simulink subsystem "sscfluids_ev_thermal_management"  (R2021b)
settings: Solver=VariableStepAuto  StartTime=0.0  StopTime=10.0  RelTol=1e-3
undefined symbols (not defined in the file): BattTempInit, bulb, cabin_duct_area, cabin_T_init, chiller_area_primary, chiller_N_baffles, chiller_N_tubes, chiller_tube_D, chiller_tube_L, chiller_wall_conductivity, chiller_wall_thickness, compressor_rpm_LUT, condenser_air_area_flow, condenser_air_area_primary, condenser_W, condenser_wall_conductivity, condenser_wall_thickness, coolant_channel_D, coolant_pipe_D, coolant_T_init, coolant_tank_area, coolant_tank_volume, coolant_valve_D_ratio_max, coolant_valve_D_ratio_min, coolant_valve_displacement, evaporator_air_area_flow, evaporator_air_area_primary, evaporator_W, evaporator_wall_conductivity, evaporator_wall_thickness, fan_area, outlet, pump_displacement, pump_speed_max, radiator_air_area_flow, radiator_air_area_primary, radiator_W, radiator_wall_conductivity, radiator_wall_thickness, refrigerant_alpha_init, refrigerant_pipe_D
libraries: fl_lib x160, nesl_utility x61, SimscapeFluids_lib x22, slpidlib x2
(part 2 of 5)

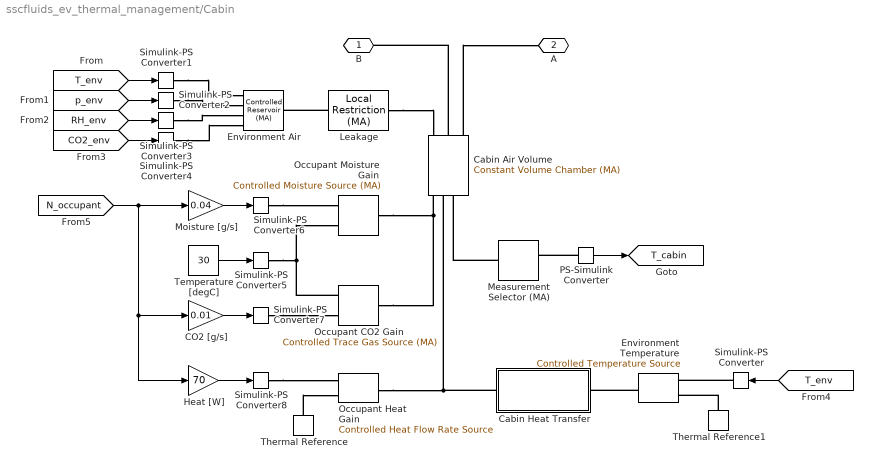
== system sscfluids_ev_thermal_management/Cabin ==
  CO2 [g/s] : Gain  Gain=0.01
  Cabin Air Volume : fl_lib/Moist Air/Elements/Constant Volume Chamber (MA)  volume=3 m^3  num_ports=foundation.enum.num_ports.three  area_A=cabin_duct_area m^2  area_B=cabin_duct_area m^2  area_C=1 m^2  area_D=0.01 m^2  RH_ws=1  time_constant=1e-3 s  moisture_trace_gas_source=foundation.enum.moisture_trace_gas_source.controlled  moisture_source_spec=foundation.enum.moisture_source_spec.vapor  moisture_mass_flow=0 kg/s  moisture_temperature_spec=foundation.enum.temperature_spec.atmospheric  moisture_temperature=293.15 K  trace_gas_mass_flow=0 kg/s  trace_gas_temperature_spec=foundation.enum.temperature_spec.atmospheric  trace_gas_temperature=293.15 K  p_I_specify=on  p_I_priority=High  p_I=cabin_p_init MPa  p_I_nominal_specify=off  p_I_nominal_unit=MPa  p_I_nominal_value=1  T_I_specify=on  T_I_priority=High  T_I=cabin_T_init degC  T_I_nominal_specify=off  T_I_nominal_unit=K  T_I_nominal_value=1  RH_I_specify=on  RH_I_priority=High  RH_I=cabin_RH_init  RH_I_nominal_specify=off  RH_I_nominal_unit=1  RH_I_nominal_value=1  x_w_I_specify=off  x_w_I_priority=None  x_w_I=0  x_w_I_nominal_specify=off  x_w_I_nominal_unit=1  x_w_I_nominal_value=1  y_w_I_specify=off  y_w_I_priority=None  y_w_I=0  y_w_I_nominal_specify=off  y_w_I_nominal_unit=1  y_w_I_nominal_value=1  HR_I_specify=off  HR_I_priority=None  HR_I=0  HR_I_nominal_specify=off  HR_I_nominal_unit=1  HR_I_nominal_value=1  x_g_I_specify=on  x_g_I_priority=None  x_g_I=0  x_g_I_nominal_specify=off  x_g_I_nominal_unit=1  x_g_I_nominal_value=1  y_g_I_specify=on  y_g_I_priority=High  y_g_I=cabin_CO2_init  y_g_I_nominal_specify=off  y_g_I_nominal_unit=1  y_g_I_nominal_value=1
      settings: SourceProductBaseCode=SS  InternalSimscapePortConfiguration="{\"Bottom\":[],\"Left\":[{\"id\":\"A\",\"label\":\"A\",\"type\":\"foundation.moist_air.moist_air\"},{\"id\":\"B\",\"label\":\"B\",\"type\":\"foundation.moist_air.moist_air\"},{\"id\":\"C\",\"label\":\"C\",\"type\":\"foundation.moist_air.moist_air\"}],\"Right\":[{\"id\":\"W\",\"label\":\"W\",\"type\":\"output\"},{\"id\":\"F\",\"label\":\"F\",\"type\":\"output\"},{\"id\":\"H\",\"label\":\"H\",\"type\":\"foundation.thermal.thermal\"},{\"id\":\"S\",\"label\":\"S\",\"type\":\"foundation.moist_air.moist_air_source\"}],\"Top\":[]}"
  Cabin Heat Transfer : Subsystem  Tag=PublishSubsystem  mask(Cabin Heat Transfer){glass_area=3.5, glass_thickness=0.004, glass_mass=3.5 * 0.004 * 2600, glass_specific_heat=840, glass_conductivity=0.96, glass_heat_coeff=40, glass_initial_temperature=cabin_T_init, doors_area=4, doors_thickness=0.06, doors_mass=75, doors_specific_heat=500, doors_conductivity=0.08, doors_heat_coeff=40, doors_initial_temperature=cabin_T_init, roof_area=2, roof_thickness=0.04, roof_mass=30, roof_specific_heat=500, roof_conductivity=0.08, roof_heat_coeff=40, roof_initial_temperature=cabin_T_init}
      mask prompts: glass_area "Area (m^2)"; glass_thickness "Thickness (m)"; glass_mass "Mass (kg)"; glass_specific_heat "Specific heat (J/kg/K)"; glass_conductivity "Thermal conductivity (W/m/K)"; glass_heat_coeff "Convective heat transfer coefficient (W/m^2/K)"; glass_initial_temperature "Initial temperature (degC)"; doors_area "Area (m^2)"; doors_thickness "Thickness (m)"; doors_mass "Mass (kg)"; doors_specific_heat "Specific heat (J/kg/K)"; doors_conductivity "Thermal conductivity (W/m/K)"; doors_heat_coeff "Convective heat transfer coefficient (W/m^2/K)"; doors_initial_temperature "Initial temperature (degC)"; roof_area "Area (m^2)"; roof_thickness "Thickness (m)"; roof_mass "Mass (kg)"; roof_specific_heat "Specific heat (J/kg/K)"; roof_conductivity "Thermal conductivity (W/m/K)"; roof_heat_coeff "Convective heat transfer coefficient (W/m^2/K)"; roof_initial_temperature "Initial temperature (degC)"
      mask DialogControl GlassTabVar Prompt: Glass
      mask DialogControl DoorsTabVar Prompt: Doors
      mask DialogControl RoofTabVar Prompt: Roof
  Environment Air : fl_lib/Moist Air/Elements/Controlled Reservoir (MA)  moisture_spec=foundation.enum.moisture_spec.relative_humidity  trace_gas_spec=foundation.enum.trace_gas_spec.mole_fraction  RH_ws=1  area_A=1 m^2  input_error_spec=foundation.enum.input_range_error.warn
      settings: SourceProductBaseCode=SS  InternalSimscapePortConfiguration="{\"Bottom\":[],\"Left\":[{\"id\":\"A\",\"label\":\"A\",\"type\":\"foundation.moist_air.moist_air\"}],\"Right\":[{\"id\":\"T\",\"label\":\"T\",\"type\":\"input\"},{\"id\":\"P\",\"label\":\"P\",\"type\":\"input\"},{\"id\":\"W\",\"label\":\"W\",\"type\":\"input\"},{\"id\":\"G\",\"label\":\"G\",\"type\":\"input\"}],\"Top\":[]}"
  Environment Temperature : fl_lib/Thermal/Thermal Sources/Controlled Temperature Source
  Heat [W] : Gain  Gain=70
  Leakage : fl_lib/Moist Air/Elements/Local Restriction (MA)  restriction_type=foundation.enum.restriction_type.fixed  restriction_area=0.004 m^2  min_area=1e-10 m^2  max_area=0.005 m^2  area=1 m^2  Cd=0.8  B_lam=0.999
      settings: SourceProductBaseCode=SS  InternalSimscapePortConfiguration="{\"Bottom\":[],\"Left\":[{\"id\":\"A\",\"label\":\"A\",\"type\":\"foundation.moist_air.moist_air\"}],\"Right\":[{\"id\":\"B\",\"label\":\"B\",\"type\":\"foundation.moist_air.moist_air\"}],\"Top\":[]}"
  Measurement Selector (MA) : fl_lib/Moist Air/Sensors/Measurement Selector (MA)  moisture_spec=foundation.enum.moisture_spec.relative_humidity  trace_gas_spec=foundation.enum.trace_gas_spec.mole_fraction
      settings: SourceProductBaseCode=SS
  Moisture [g/s] : Gain  Gain=0.04
  Occupant CO2 Gain : fl_lib/Moist Air/Sources/Moisture & Trace Gas Sources/Controlled Trace Gas Source (MA)  Phi_S_specify=off  Phi_S_priority=None  Phi_S=0 kW  Phi_S_nominal_specify=off  Phi_S_nominal_unit=kW  Phi_S_nominal_value=1  mdot_g_S_specify=off  mdot_g_S_priority=None  mdot_g_S=0 kg/s  mdot_g_S_nominal_specify=off  mdot_g_S_nominal_unit=kg/s  mdot_g_S_nominal_value=1
      settings: SourceProductBaseCode=SS  InternalSimscapePortConfiguration="{\"Bottom\":[],\"Left\":[{\"id\":\"S\",\"label\":\"S\",\"type\":\"foundation.moist_air.moist_air_source\"}],\"Right\":[{\"id\":\"M\",\"label\":\"M\",\"type\":\"input\"},{\"id\":\"T\",\"label\":\"T\",\"type\":\"input\"}],\"Top\":[]}"
  Occupant Heat Gain : fl_lib/Thermal/Thermal Sources/Controlled Heat Flow Rate Source
  Occupant Moisture Gain : fl_lib/Moist Air/Sources/Moisture & Trace Gas Sources/Controlled Moisture Source (MA)  moisture_source_spec=foundation.enum.moisture_source_spec.vapor  Phi_S_specify=off  Phi_S_priority=None  Phi_S=0 kW  Phi_S_nominal_specify=off  Phi_S_nominal_unit=kW  Phi_S_nominal_value=1  mdot_w_S_specify=off  mdot_w_S_priority=None  mdot_w_S=0 kg/s  mdot_w_S_nominal_specify=off  mdot_w_S_nominal_unit=kg/s  mdot_w_S_nominal_value=1
      settings: SourceProductBaseCode=SS  InternalSimscapePortConfiguration="{\"Bottom\":[],\"Left\":[{\"id\":\"S\",\"label\":\"S\",\"type\":\"foundation.moist_air.moist_air_source\"}],\"Right\":[{\"id\":\"M\",\"label\":\"M\",\"type\":\"input\"},{\"id\":\"T\",\"label\":\"T\",\"type\":\"input\"}],\"Top\":[]}"
  PS-Simulink Converter : nesl_utility/PS-Simulink Converter  PhysicalDomain=network_engine_domain  SubClassName=ps_output  LeftPortType=input  RightPortType=output  PseudoPeriodic=off  Frequencies=[]  Unit=degC  AffineConversion=on
      settings: SourceProductBaseCode=PW,SS
  Simulink-PS Converter : nesl_utility/Simulink-PS Converter  PhysicalDomain=network_engine_domain  SubClassName=ps_input  LeftPortType=input  RightPortType=output  PseudoPeriodic=off  Frequencies=[]  NoiseDistribution=none  NoiseParameters=[]  Unit=degC  AffineConversion=on  FilteringAndDerivatives=provide  SimscapeFilterOrder=1  InputFilterTimeConstant=0.001  UdotUserProvided=0
      settings: SourceProductBaseCode=PW,SS
  Simulink-PS Converter1 : nesl_utility/Simulink-PS Converter  PhysicalDomain=network_engine_domain  SubClassName=ps_input  LeftPortType=input  RightPortType=output  PseudoPeriodic=off  Frequencies=[]  NoiseDistribution=none  NoiseParameters=[]  Unit=degC  AffineConversion=on  FilteringAndDerivatives=provide  SimscapeFilterOrder=1  InputFilterTimeConstant=0.001  UdotUserProvided=0
      settings: SourceProductBaseCode=PW,SS
  Simulink-PS Converter2 : nesl_utility/Simulink-PS Converter  PhysicalDomain=network_engine_domain  SubClassName=ps_input  LeftPortType=input  RightPortType=output  PseudoPeriodic=off  Frequencies=[]  NoiseDistribution=none  NoiseParameters=[]  Unit=MPa  AffineConversion=off  FilteringAndDerivatives=provide  SimscapeFilterOrder=1  InputFilterTimeConstant=0.001  UdotUserProvided=0
      settings: SourceProductBaseCode=PW,SS
  Simulink-PS Converter3 : nesl_utility/Simulink-PS Converter  PhysicalDomain=network_engine_domain  SubClassName=ps_input  LeftPortType=input  RightPortType=output  PseudoPeriodic=off  Frequencies=[]  NoiseDistribution=none  NoiseParameters=[]  Unit=1  AffineConversion=off  FilteringAndDerivatives=provide  SimscapeFilterOrder=1  InputFilterTimeConstant=0.001  UdotUserProvided=0
      settings: SourceProductBaseCode=PW,SS
  Simulink-PS Converter4 : nesl_utility/Simulink-PS Converter  PhysicalDomain=network_engine_domain  SubClassName=ps_input  LeftPortType=input  RightPortType=output  PseudoPeriodic=off  Frequencies=[]  NoiseDistribution=none  NoiseParameters=[]  Unit=1  AffineConversion=off  FilteringAndDerivatives=provide  SimscapeFilterOrder=1  InputFilterTimeConstant=0.001  UdotUserProvided=0
      settings: SourceProductBaseCode=PW,SS
  Simulink-PS Converter5 : nesl_utility/Simulink-PS Converter  PhysicalDomain=network_engine_domain  SubClassName=ps_input  LeftPortType=input  RightPortType=output  PseudoPeriodic=off  Frequencies=[]  NoiseDistribution=none  NoiseParameters=[]  Unit=degC  AffineConversion=on  FilteringAndDerivatives=provide  SimscapeFilterOrder=1  InputFilterTimeConstant=0.001  UdotUserProvided=0
      settings: SourceProductBaseCode=PW,SS
  Simulink-PS Converter6 : nesl_utility/Simulink-PS Converter  PhysicalDomain=network_engine_domain  SubClassName=ps_input  LeftPortType=input  RightPortType=output  PseudoPeriodic=off  Frequencies=[]  NoiseDistribution=none  NoiseParameters=[]  Unit=g/s  AffineConversion=off  FilteringAndDerivatives=provide  SimscapeFilterOrder=1  InputFilterTimeConstant=0.001  UdotUserProvided=0
      settings: SourceProductBaseCode=PW,SS
  Simulink-PS Converter7 : nesl_utility/Simulink-PS Converter  PhysicalDomain=network_engine_domain  SubClassName=ps_input  LeftPortType=input  RightPortType=output  PseudoPeriodic=off  Frequencies=[]  NoiseDistribution=none  NoiseParameters=[]  Unit=g/s  AffineConversion=off  FilteringAndDerivatives=provide  SimscapeFilterOrder=1  InputFilterTimeConstant=0.001  UdotUserProvided=0
      settings: SourceProductBaseCode=PW,SS
  Simulink-PS Converter8 : nesl_utility/Simulink-PS Converter  PhysicalDomain=network_engine_domain  SubClassName=ps_input  LeftPortType=input  RightPortType=output  PseudoPeriodic=off  Frequencies=[]  NoiseDistribution=none  NoiseParameters=[]  Unit=W  AffineConversion=off  FilteringAndDerivatives=provide  SimscapeFilterOrder=1  InputFilterTimeConstant=0.001  UdotUserProvided=0
      settings: SourceProductBaseCode=PW,SS
  Temperature [degC] : Constant  Value=30
  Thermal Reference : fl_lib/Thermal/Thermal Elements/Thermal Reference
  Thermal Reference1 : fl_lib/Thermal/Thermal Elements/Thermal Reference
  B : PMIOPort  Side=Left
  A : PMIOPort  Port=2  Side=Right
  tag scope: T_cabin=global
  wires:
  PS-Simulink Converter/1 -> [T_cabin]
  [T_env] -> Simulink-PS Converter1/1
  [p_env] -> Simulink-PS Converter2/1
  [RH_env] -> Simulink-PS Converter3/1
  [CO2_env] -> Simulink-PS Converter4/1
  [T_env] -> Simulink-PS Converter/1
  Moisture [g/s]/1 -> Simulink-PS Converter6/1
  CO2 [g/s]/1 -> Simulink-PS Converter7/1
  Heat [W]/1 -> Simulink-PS Converter8/1
  [N_occupant] -> Moisture [g/s]/1, CO2 [g/s]/1, Heat [W]/1
  Temperature [degC]/1 -> Simulink-PS Converter5/1
  connections:
  Cabin Air Volume/LConn1 -- A/RConn1
  Cabin Air Volume/LConn2 -- B/RConn1
  Simulink-PS Converter3/RConn1 -- Environment Air/RConn3
  Simulink-PS Converter4/RConn1 -- Environment Air/RConn4
  Simulink-PS Converter2/RConn1 -- Environment Air/RConn2
  Simulink-PS Converter1/RConn1 -- Environment Air/RConn1
  Leakage/RConn1 -- Environment Air/LConn1
  Leakage/LConn1 -- Cabin Air Volume/LConn3
  Occupant Moisture Gain/LConn1 -- Occupant CO2 Gain/LConn1 -- Cabin Air Volume/RConn4
  Occupant Heat Gain/LConn1 -- Cabin Air Volume/RConn3 -- Cabin Heat Transfer/LConn1
  Thermal Reference/LConn1 -- Occupant Heat Gain/RConn2
  Simulink-PS Converter5/RConn1 -- Occupant CO2 Gain/RConn2 -- Occupant Moisture Gain/RConn2
  Simulink-PS Converter6/RConn1 -- Occupant Moisture Gain/RConn1
  Simulink-PS Converter7/RConn1 -- Occupant CO2 Gain/RConn1
  Simulink-PS Converter8/RConn1 -- Occupant Heat Gain/RConn1
  Environment Temperature/LConn1 -- Cabin Heat Transfer/RConn1
  Thermal Reference1/LConn1 -- Environment Temperature/RConn2
  Simulink-PS Converter/RConn1 -- Environment Temperature/RConn1
  Measurement Selector (MA)/LConn1 -- Cabin Air Volume/RConn2
  PS-Simulink Converter/LConn1 -- Measurement Selector (MA)/RConn2

== system sscfluids_ev_thermal_management/Chiller ==
  Chiller : SimscapeFluids_lib/Fluid Network Interfaces/Heat Exchangers/Condenser Evaporator (TL-2P)  flow_arrangement=fluids.interfaces.heat_exchangers.enum.FlowArrangementTL2P.Cross  cross_flow_arrangement=fluids.interfaces.heat_exchangers.enum.CrossFlowArrangementTL2P.UnmixedMixed  R_wall=chiller_wall_thickness / chiller_area_primary / chiller_wall_conductivity K/kW  area_A1=pi * coolant_pipe_D^2 / 4 m^2  area_B1=pi * coolant_pipe_D^2 / 4 m^2  area_A2=pi * refrigerant_pipe_D^2 / 4 m^2  area_B2=pi * refrigerant_pipe_D^2 / 4 m^2  flow_geometry_TL=fluids.interfaces.heat_exchangers.enum.FlowGeometryTL.AcrossTubeBank  tube_num_TL=1  tube_length_TL=5 m  tube_cross_section_TL=fluids.interfaces.heat_exchangers.enum.TubeCrossSection.Circular  tube_diameter_TL=0.1 m  tube_width_TL=0.1 m  tube_height_TL=0.1 m  tube_inner_diameter_TL=0.05 m  tube_outer_diameter_TL=0.1 m  tube_flow_area_TL=0.01 m^2  tube_wetted_perimeter_TL=0.4 m  tube_heat_perimeter_TL=0.4 m  tube_pressure_loss_spec_TL=fluids.interfaces.heat_exchangers.enum.TubePressureLossSpec.Haaland  tube_loss_coeff_TL=10  tube_length_add_TL=0.1 m  tube_roughness_pressure_TL=15e-6 m  tube_Re_lam_pressure_TL=2000  tube_Re_tur_pressure_TL=4000  tube_shape_factor_generic_TL=64  tube_heat_coeff_spec_TL=fluids.interfaces.heat_exchangers.enum.TubeHeatCoeffSpec.Gneilinski  tube_colburn_coeff_TL=[.023, .8, .33]  tube_roughness_heat_TL=15e-6 m  tube_Re_lam_heat_TL=2000  tube_Re_tur_heat_TL=4000  tube_Nu_lam_generic_TL=3.66  bank_arrangement_TL=fluids.interfaces.heat_exchangers.enum.BankArrangement.Staggered  bank_num_rows_TL=sqrt(chiller_N_tubes) * (chiller_N_baffles + 1)  bank_tubes_per_row_TL=sqrt(chiller_N_tubes)  bank_width_TL=chiller_tube_L / (chiller_N_baffles + 1) m  bank_tube_diameter_TL=chiller_tube_D m  bank_longitudinal_pitch_TL=2 * chiller_tube_D m  bank_transverse_pitch_TL=2 * chiller_tube_D m  bank_pressure_loss_spec_TL=fluids.interfaces.heat_exchangers.enum.BankPressureLossSpec.Martin  bank_euler_TL=10  bank_heat_coeff_spec_TL=fluids.interfaces.heat_exchangers.enum.BankHeatCoeffSpec.Martin  bank_colburn_coeff_TL=[.27, .63, .36]  generic_flow_area_TL=0.01 m^2  generic_heat_area_TL=2 m^2  generic_volume_TL=0.05 m^3  generic_loss_coeff_TL=10  generic_colburn_coeff_TL=[.023, .8, .33]  fouling_factor_TL=0.1 m^2*K/kW  fin_area_TL=chiller_area_baffles m^2  fin_efficiency_TL=0.5  p_init_TL=coolant_p_init MPa  T_init_TL=coolant_T_init degC  tube_num_2P=chiller_N_tubes  tube_length_2P=chiller_tube_L m  tube_cross_section_2P=fluids.interfaces.heat_exchangers.enum.TubeCrossSection.Circular  tube_diameter_2P=chiller_tube_D m  tube_width_2P=0.1 m  tube_height_2P=0.1 m  tube_inner_diameter_2P=0.05 m  tube_outer_diameter_2P=0.1 m  tube_flow_area_2P=0.01 m^2  tube_wetted_perimeter_2P=0.4 m  tube_heat_perimeter_2P=0.4 m  tube_pressure_loss_spec_2P=fluids.interfaces.heat_exchangers.enum.TubePressureLossSpec2P.Haaland  tube_loss_coeff_2P=10  tube_length_add_2P=chiller_tube_Leq m  tube_roughness_pressure_2P=15e-6 m  tube_Re_lam_pressure_2P=2000  tube_Re_tur_pressure_2P=4000  tube_shape_factor_generic_2P=64  tube_heat_coeff_spec_2P=fluids.interfaces.heat_exchangers.enum.TubeHeatCoeffSpec2P.GneilinskiCavalliniZecchin  tube_colburn_coeff_liq_2P=[.023, .8, .33]  tube_colburn_coeff_mix_2P=[.05, .8, .33]  tube_colburn_coeff_vap_2P=[.023, .8, .33]  tube_roughness_heat_2P=15e-6 m  tube_Re_lam_heat_2P=2000  tube_Re_tur_heat_2P=4000  tube_Nu_lam_generic_2P=3.66  fouling_factor_2P=0.1 m^2*K/kW  fin_area_2P=0 m^2  fin_efficiency_2P=0  energy_spec_2P=foundation.enum.energy_spec.void_fraction  p_init_2P=refrigerant_p_init MPa  T_init_2P=293.15 K  x_init_2P=0.5  alpha_init_2P=refrigerant_alpha_init  h_init_2P=1500 kJ/kg  u_init_2P=1500 kJ/kg
      settings: SourceProductBaseCode=SH  InternalSimscapePortConfiguration="{\"Bottom\":[],\"Left\":[{\"id\":\"A1\",\"label\":\"A1\",\"type\":\"foundation.thermal_liquid.thermal_liquid\"},{\"id\":\"B1\",\"label\":\"B1\",\"type\":\"foundation.thermal_liquid.thermal_liquid\"}],\"Right\":[{\"id\":\"A2\",\"label\":\"A2\",\"type\":\"foundation.two_phase_fluid.two_phase_fluid\"},{\"id\":\"B2\",\"label\":\"B2\",\"type\":\"foundation.two_phase_fluid.two_phase_fluid\"}],\"Top\":[{\"id\":\"Z\",\"label\":\"Z\",\"type\":\"output\"}]}"
  Flow Resistance (2P) : fl_lib/Two-Phase Fluid/Elements/Flow Resistance (2P)  delta_p_nominal=1e-4 MPa  mdot_nominal=0.01 kg/s  v_nominal=0 m^3/kg  area=pi * refrigerant_pipe_D^2 / 4 m^2  laminar_fraction=1e-3
      settings: SourceProductBaseCode=SS  InternalSimscapePortConfiguration="{\"Bottom\":[],\"Left\":[{\"id\":\"A\",\"label\":\"A\",\"type\":\"foundation.two_phase_fluid.two_phase_fluid\"}],\"Right\":[{\"id\":\"B\",\"label\":\"B\",\"type\":\"foundation.two_phase_fluid.two_phase_fluid\"}],\"Top\":[]}"
  SR3 : Subsystem
      mask Display: disp(get_param(gcb, 'Name'))
  SR4 : Subsystem
      mask Display: disp(get_param(gcb, 'Name'))
  Simscape Bus : SimscapeBus  HierarchyStrings=bulb;outlet
  B : PMIOPort  Side=Left
  A : PMIOPort  Port=2  Side=Right
  C : PMIOPort  Port=3  Side=Left
  D : PMIOPort  Port=4  Side=Right
  connections:
  Chiller/LConn2 -- C/RConn1
  Chiller/LConn1 -- D/RConn1
  Chiller/RConn1 -- SR3/LConn1
  SR4/RConn1 -- Chiller/RConn2 -- Simscape Bus/LConn1
  Simscape Bus/LConn2 -- SR3/RConn1
  A/RConn1 -- Simscape Bus/RConn1
  B/RConn1 -- Flow Resistance (2P)/RConn1
  Flow Resistance (2P)/LConn1 -- SR4/LConn1

== system sscfluids_ev_thermal_management/Chiller Bypass Valve ==
  Bias : Bias  Bias=-1
  Chiller Bypass Valve : SimscapeFluids_lib/Thermal Liquid/Valves & Orifices/Directional Control Valves/3-Way Directional Valve (TL)  area_spec=fluids.thermal_liquid.valves.directional_control_valves.enum.area_spec.identical  valve_spec_identical=fluids.thermal_liquid.valves.enum.orifice_spec.linear  valve_spec_different=fluids.thermal_liquid.valves.enum.orifice_spec.linear  area_leak=pi * (coolant_valve_D_ratio_min*coolant_pipe_D)^2 / 4 m^2  area=pi * coolant_pipe_D^2 / 4 m^2  length=0.05 m  Cd=0.7  Re_c=12  opening_max=coolant_valve_displacement m  area_max=pi * (coolant_valve_D_ratio_max*coolant_pipe_D)^2 / 4 m^2  opening_TLU=[-.002, 0, .002, .005, .015] m  valve_area_TLU=[1e-09, 2.0352e-07, 4.0736e-05, .00011438, .00034356] m^2  opening_mdot_TLU=[-.002, 0, .002, .005, .015] m  p_diff_TLU=[-.1, .3, .5, .7] MPa  mdot_TLU=[-1e-05, 1.7e-05, 2e-05, 2.6e-05; -.002, .0035, .0045, .0053; -.4, .7, .9, 1.06; -1.13, 1.96, 2.5, 3; -3.45, 6, 7.7, 9.13] kg/s  T_ref_in=293.15 K  p_ref_in=0.101325 MPa  opening_max_P=0.005 m  area_max_P=1e-4 m^2  opening_TLU_P=[-.002, 0, .002, .005, .015] m  valve_area_TLU_P=[1e-09, 2.0352e-07, 4.0736e-05, .00011438, .00034356] m^2  opening_mdot_TLU_P=[-.002, 0, .002, .005, .015] m  p_diff_TLU_P=[-.1, .3, .5, .7] MPa  mdot_TLU_P=[-1e-05, 1.7e-05, 2e-05, 2.6e-05; -.002, .0035, .0045, .0053; -.4, .7, .9, 1.06; -1.13, 1.96, 2.5, 3; -3.45, 6, 7.7, 9.13] kg/s  T_ref_in_P=293.15 K  p_ref_in_P=0.101325 MPa  opening_max_T=0.005 m  area_max_T=1e-4 m^2  opening_TLU_T=[-.002, 0, .002, .005, .015] m  valve_area_TLU_T=[1e-09, 2.0352e-07, 4.0736e-05, .00011438, .00034356] m^2  opening_mdot_TLU_T=[-.002, 0, .002, .005, .015] m  p_diff_TLU_T=[-.1, .3, .5, .7] MPa  mdot_TLU_T=[-1e-05, 1.7e-05, 2e-05, 2.6e-05; -.002, .0035, .0045, .0053; -.4, .7, .9, 1.06; -1.13, 1.96, 2.5, 3; -3.45, 6, 7.7, 9.13] kg/s  T_ref_in_T=293.15 K  p_ref_in_T=0.101325 MPa  smoothing_factor=0.01  x0_P=coolant_valve_offset m  x0_T=coolant_valve_offset m
      settings: SourceProductBaseCode=SH  InternalSimscapePortConfiguration="{\"Bottom\":[],\"Left\":[{\"id\":\"A\",\"label\":\"A\",\"type\":\"foundation.thermal_liquid.thermal_liquid\"}],\"Right\":[{\"id\":\"S\",\"label\":\"S\",\"type\":\"input\"},{\"id\":\"P\",\"label\":\"P\",\"type\":\"foundation.thermal_liquid.thermal_liquid\"},{\"id\":\"T\",\"label\":\"T\",\"type\":\"foundation.thermal_liquid.thermal_liquid\"}],\"Top\":[]}"
  Flow Resistance (TL) : fl_lib/Thermal Liquid/Elements/Flow Resistance (TL)  delta_p_nominal=0.001 MPa  mdot_nominal=0.3 kg/s  area=pi * coolant_pipe_D^2 / 4 m^2  laminar_fraction=1e-3
      settings: SourceProductBaseCode=SS
  Gain : Gain  Gain=2
  Max Valve Displacement [m] : Gain  Gain=coolant_valve_displacement
  Simulink-PS Converter : nesl_utility/Simulink-PS Converter  PhysicalDomain=network_engine_domain  SubClassName=ps_input  LeftPortType=input  RightPortType=output  PseudoPeriodic=off  Frequencies=[]  NoiseDistribution=none  NoiseParameters=[]  Unit=m  AffineConversion=off  FilteringAndDerivatives=provide  SimscapeFilterOrder=1  InputFilterTimeConstant=0.001  UdotUserProvided=0
      settings: SourceProductBaseCode=PW,SS
  Transfer Fcn : TransferFcn  Denominator=[1 1]
  A : PMIOPort  Side=Left
  C : PMIOPort  Port=2  Side=Left
  B : PMIOPort  Port=3  Side=Right
  wires:
  Max Valve Displacement [m]/1 -> Simulink-PS Converter/1
  Bias/1 -> Max Valve Displacement [m]/1
  Gain/1 -> Bias/1
  Transfer Fcn/1 -> Gain/1
  [cmd_chiller_bypass] -> Transfer Fcn/1
  connections:
  A/RConn1 -- Chiller Bypass Valve/LConn1
  C/RConn1 -- Chiller Bypass Valve/RConn3
  Simulink-PS Converter/RConn1 -- Chiller Bypass Valve/RConn1
  Flow Resistance (TL)/LConn1 -- Chiller Bypass Valve/RConn2
  Flow Resistance (TL)/RConn1 -- B/RConn1

== system sscfluids_ev_thermal_management/Chiller Expansion Valve ==
  Chiller Expansion Valve : SimscapeFluids_lib/Two-Phase Fluid/Valves & Orifices/Flow Control Valves/Thermostatic Expansion Valve (2P)  Q_nominal=4500 W  Q_max=7000 W  T_evap=1 degC  delta_T_static=5 degC  delta_T_nominal=10 degC  T_cond=40 degC  delta_T_sub=5 degC  pressure_equalization=fluids.two_phase_fluid.valves_orifices.flow_control_valves.enum.ThermostaticExpansionValveEqualization.External  mop=fluids.two_phase_fluid.valves_orifices.flow_control_valves.enum.ThermostaticExpansionValveMOP.Off  p_mop=0.5 MPa  T_mop=288.15 K  bulb_dynamics=simscape.enum.onoff.off  tau_bulb=20 s  area=pi * refrigerant_pipe_D^2 / 4 m^2  mdot_leak_fraction=1e-4  smoothing_factor=0.01  B_lam=0.999  tau_x=0.1 s
      settings: SourceProductBaseCode=SH  InternalSimscapePortConfiguration="{\"Bottom\":[],\"Left\":[{\"id\":\"A\",\"label\":\"A\",\"type\":\"foundation.two_phase_fluid.two_phase_fluid\"}],\"Right\":[{\"id\":\"B\",\"label\":\"B\",\"type\":\"foundation.two_phase_fluid.two_phase_fluid\"}],\"Top\":[{\"id\":\"S\",\"label\":\"S\",\"type\":\"foundation.two_phase_fluid.two_phase_fluid\"},{\"id\":\"E\",\"label\":\"E\",\"type\":\"foundation.two_phase_fluid.two_phase_fluid\"}]}"
  Simscape Bus : SimscapeBus  HierarchyStrings=bulb;outlet
  B : PMIOPort  Side=Left
  A : PMIOPort  Port=2  Side=Right
  connections:
  A/RConn1 -- Chiller Expansion Valve/LConn1
  Simscape Bus/LConn2 -- Chiller Expansion Valve/RConn1
  Chiller Expansion Valve/LConn3 -- Chiller Expansion Valve/LConn2 -- Simscape Bus/LConn1
  Simscape Bus/RConn1 -- B/RConn1

== system sscfluids_ev_thermal_management/Compressor ==
  Compressor : fl_lib/Two-Phase Fluid/Sources/Controlled Mass Flow Rate Source (2P)  power_spec=foundation.enum.power_spec.isentropic  area_A=pi * refrigerant_pipe_D^2 / 4 m^2  area_B=pi * refrigerant_pipe_D^2 / 4 m^2
      settings: SourceProductBaseCode=SS  InternalSimscapePortConfiguration="{\"Bottom\":[],\"Left\":[{\"id\":\"A\",\"label\":\"A\",\"type\":\"foundation.two_phase_fluid.two_phase_fluid\"},{\"id\":\"M\",\"label\":\"M\",\"type\":\"input\"}],\"Right\":[{\"id\":\"B\",\"label\":\"B\",\"type\":\"foundation.two_phase_fluid.two_phase_fluid\"}],\"Top\":[]}"
  Compressor Map : Subsystem
  Max Speed [rpm] : Gain  Gain=max(compressor_rpm_LUT)
  Simulink-PS Converter : nesl_utility/Simulink-PS Converter  PhysicalDomain=network_engine_domain  SubClassName=ps_input  LeftPortType=input  RightPortType=output  PseudoPeriodic=off  Frequencies=[]  NoiseDistribution=none  NoiseParameters=[]  Unit=rpm  AffineConversion=off  FilteringAndDerivatives=provide  SimscapeFilterOrder=1  InputFilterTimeConstant=0.001  UdotUserProvided=0
      settings: SourceProductBaseCode=PW,SS
  Transfer Fcn : TransferFcn  Denominator=[5 1]
  B : PMIOPort  Side=Left
  A : PMIOPort  Port=2  Side=Right
  wires:
  Max Speed [rpm]/1 -> Simulink-PS Converter/1
  Transfer Fcn/1 -> Max Speed [rpm]/1
  [cmd_comp] -> Transfer Fcn/1
  connections:
  Compressor/LConn1 -- A/RConn1 -- Compressor Map/RConn1
  Compressor/RConn1 -- B/RConn1 -- Compressor Map/RConn3
  Compressor Map/RConn2 -- Simulink-PS Converter/RConn1
  Compressor/LConn2 -- Compressor Map/LConn1

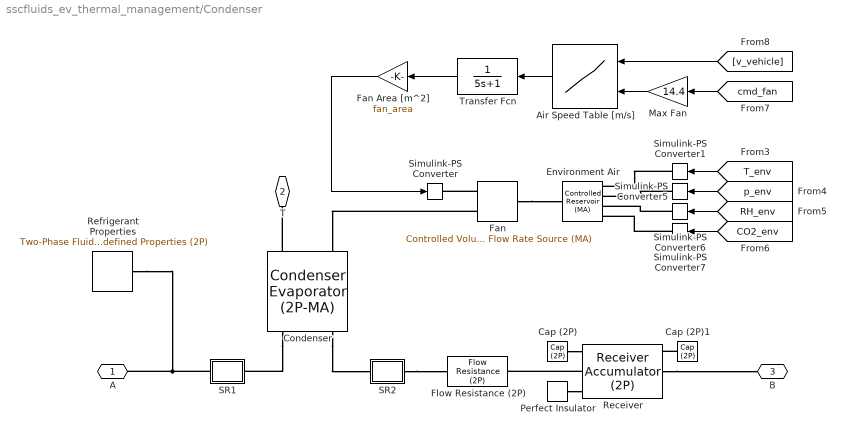
== system sscfluids_ev_thermal_management/Condenser ==
  Air Speed Table [m/s] : Lookup_n-D  BreakpointsForDimension1=[0 40 90 110 150 180 198]  BreakpointsForDimension2=[0 14.4]  IndexSearchMethod=Linear search  BeginIndexSearchUsingPreviousIndexResult=on  Table=[0 0.8 2.2 2.7 3.6 4.1 4.6; 1.5 2.3 3.2 3.5 4.3 4.8 5.1]'  InternalRulePriority=Speed  RndMeth=Simplest  InputSameDT=on
      settings: InputPortMap=u0,u1
  Cap (2P) : fl_lib/Two-Phase Fluid/Elements/Cap (2P)  p_specify=off  p_priority=None  p=0.101325 MPa  p_nominal_specify=off  p_nominal_unit=MPa  p_nominal_value=1  u_specify=off  u_priority=None  u=1.5e+3 kJ/kg  u_nominal_specify=off  u_nominal_unit=kJ/kg  u_nominal_value=1
      settings: SourceProductBaseCode=SS  InternalSimscapePortConfiguration="{\"Bottom\":[],\"Left\":[{\"id\":\"A\",\"label\":\"\",\"type\":\"foundation.two_phase_fluid.two_phase_fluid\"}],\"Right\":[],\"Top\":[]}"
  Cap (2P)1 : fl_lib/Two-Phase Fluid/Elements/Cap (2P)  p_specify=off  p_priority=None  p=0.101325 MPa  p_nominal_specify=off  p_nominal_unit=MPa  p_nominal_value=1  u_specify=off  u_priority=None  u=1.5e+3 kJ/kg  u_nominal_specify=off  u_nominal_unit=kJ/kg  u_nominal_value=1
      settings: SourceProductBaseCode=SS  InternalSimscapePortConfiguration="{\"Bottom\":[],\"Left\":[{\"id\":\"A\",\"label\":\"\",\"type\":\"foundation.two_phase_fluid.two_phase_fluid\"}],\"Right\":[],\"Top\":[]}"
  Condenser : SimscapeFluids_lib/Fluid Network Interfaces/Heat Exchangers/Condenser Evaporator (2P-MA)  flow_arrangement=fluids.interfaces.heat_exchangers.enum.FlowArrangement2PMA.Cross  cross_flow_arrangement=fluids.interfaces.heat_exchangers.enum.CrossFlowArrangement2PMA.UnmixedUnmixed  R_wall=condenser_wall_thickness / condenser_air_area_primary / condenser_wall_conductivity K/kW  area_A1=pi * refrigerant_pipe_D^2 / 4 m^2  area_B1=pi * refrigerant_pipe_D^2 / 4 m^2  area_A2=cabin_duct_area m^2  area_B2=cabin_duct_area m^2  tube_num_2P=condenser_N_tubes  tube_length_2P=condenser_L m  tube_cross_section_2P=fluids.interfaces.heat_exchangers.enum.TubeCrossSection.Rectangular  tube_diameter_2P=0.1 m  tube_width_2P=condenser_W m  tube_height_2P=condenser_tube_H m  tube_inner_diameter_2P=0.05 m  tube_outer_diameter_2P=0.1 m  tube_flow_area_2P=0.01 m^2  tube_wetted_perimeter_2P=0.4 m  tube_heat_perimeter_2P=0.4 m  tube_pressure_loss_spec_2P=fluids.interfaces.heat_exchangers.enum.TubePressureLossSpec2P.Haaland  tube_loss_coeff_2P=10  tube_length_add_2P=condenser_tube_Leq m  tube_roughness_pressure_2P=15e-6 m  tube_Re_lam_pressure_2P=2000  tube_Re_tur_pressure_2P=4000  tube_shape_factor_generic_2P=64  tube_heat_coeff_spec_2P=fluids.interfaces.heat_exchangers.enum.TubeHeatCoeffSpec2P.GneilinskiCavalliniZecchin  tube_colburn_coeff_liq_2P=[.023, .8, .33]  tube_colburn_coeff_mix_2P=[.05, .8, .33]  tube_colburn_coeff_vap_2P=[.023, .8, .33]  tube_roughness_heat_2P=15e-6 m  tube_Re_lam_heat_2P=2000  tube_Re_tur_heat_2P=4000  tube_Nu_lam_generic_2P=3.66  fouling_factor_2P=0.1 m^2*K/kW  fin_area_2P=condenser_tube_area_webs m^2  fin_efficiency_2P=0.6  energy_spec_2P=foundation.enum.energy_spec.void_fraction  p_init_2P=refrigerant_p_init MPa  T_init_2P=293.15 K  x_init_2P=0.5  alpha_init_2P=refrigerant_alpha_init  h_init_2P=1500 kJ/kg  u_init_2P=1500 kJ/kg  flow_geometry_MA=fluids.interfaces.heat_exchangers.enum.FlowGeometryMA.Generic  tube_num_MA=1  tube_length_MA=5 m  tube_cross_section_MA=fluids.interfaces.heat_exchangers.enum.TubeCrossSection.Circular  tube_diameter_MA=0.1 m  tube_width_MA=0.1 m  tube_height_MA=0.1 m  tube_inner_diameter_MA=0.05 m  tube_outer_diameter_MA=0.1 m  tube_flow_area_MA=0.01 m^2  tube_wetted_perimeter_MA=0.4 m  tube_heat_perimeter_MA=0.4 m  tube_pressure_loss_spec_MA=fluids.interfaces.heat_exchangers.enum.TubePressureLossSpec.Haaland  tube_loss_coeff_MA=10  tube_length_add_MA=0.1 m  tube_roughness_pressure_MA=15e-6 m  tube_Re_lam_pressure_MA=2000  tube_Re_tur_pressure_MA=4000  tube_shape_factor_generic_MA=64  tube_heat_coeff_spec_MA=fluids.interfaces.heat_exchangers.enum.TubeHeatCoeffSpec.Gneilinski  tube_colburn_coeff_MA=[.023, .8, .33]  tube_roughness_heat_MA=15e-6 m  tube_Re_lam_heat_MA=2000  tube_Re_tur_heat_MA=4000  tube_Nu_lam_generic_MA=3.66  bank_arrangement_MA=fluids.interfaces.heat_exchangers.enum.BankArrangement.Inline  bank_num_rows_MA=5  bank_tubes_per_row_MA=5  bank_width_MA=1 m  bank_tube_diameter_MA=0.05 m  bank_longitudinal_pitch_MA=0.15 m  bank_transverse_pitch_MA=0.15 m  bank_pressure_loss_spec_MA=fluids.interfaces.heat_exchangers.enum.BankPressureLossSpec.Martin  bank_euler_MA=10  bank_heat_coeff_spec_MA=fluids.interfaces.heat_exchangers.enum.BankHeatCoeffSpec.Martin  bank_colburn_coeff_MA=[.27, .63, .36]  generic_flow_area_MA=condenser_air_area_flow m^2  generic_heat_area_MA=condenser_air_area_primary m^2  generic_volume_MA=condenser_air_area_flow * condenser_W m^3  generic_loss_coeff_MA=10  generic_colburn_coeff_MA=[0.27, 0.63, 0.36]  fouling_factor_MA=0.1 m^2*K/kW  fin_area_MA=condenser_air_area_fins m^2  fin_efficiency_MA=0.7  p_init_MA=cabin_p_init MPa  T_init_MA=cabin_T_init degC  moisture_spec_MA=foundation.enum.moisture_spec.relative_humidity  RH_init_MA=cabin_RH_init  x_w_init_MA=0.01  y_w_init_MA=0.01  HR_init_MA=0.01  trace_gas_spec_MA=foundation.enum.trace_gas_spec.mole_fraction  x_g_init_MA=0.001  y_g_init_MA=cabin_CO2_init  RH_ws_MA=1
      settings: SourceProductBaseCode=SH  InternalSimscapePortConfiguration="{\"Bottom\":[],\"Left\":[{\"id\":\"A1\",\"label\":\"A1\",\"type\":\"foundation.two_phase_fluid.two_phase_fluid\"},{\"id\":\"Z\",\"label\":\"Z\",\"type\":\"output\"},{\"id\":\"B1\",\"label\":\"B1\",\"type\":\"foundation.two_phase_fluid.two_phase_fluid\"}],\"Right\":[{\"id\":\"A2\",\"label\":\"A2\",\"type\":\"foundation.moist_air.moist_air\"},{\"id\":\"W\",\"label\":\"W\",\"type\":\"output\"},{\"id\":\"B2\",\"label\":\"B2\",\"type\":\"foundation.moist_air.moist_air\"}],\"Top\":[]}"
  Environment Air : fl_lib/Moist Air/Elements/Controlled Reservoir (MA)  moisture_spec=foundation.enum.moisture_spec.relative_humidity  trace_gas_spec=foundation.enum.trace_gas_spec.mole_fraction  RH_ws=1  area_A=cabin_duct_area m^2  input_error_spec=foundation.enum.input_range_error.warn
      settings: SourceProductBaseCode=SS  InternalSimscapePortConfiguration="{\"Bottom\":[],\"Left\":[{\"id\":\"A\",\"label\":\"A\",\"type\":\"foundation.moist_air.moist_air\"}],\"Right\":[{\"id\":\"T\",\"label\":\"T\",\"type\":\"input\"},{\"id\":\"P\",\"label\":\"P\",\"type\":\"input\"},{\"id\":\"W\",\"label\":\"W\",\"type\":\"input\"},{\"id\":\"G\",\"label\":\"G\",\"type\":\"input\"}],\"Top\":[]}"
  Fan : fl_lib/Moist Air/Sources/Controlled Volumetric Flow Rate Source (MA)  power_spec=foundation.enum.power_spec.isentropic  volumetric_flow_conditions=foundation.enum.volumetric_flow_conditions.actual  p_std=0.101325 MPa  T_std=20 degC  RH_std=0.65  area_A=cabin_duct_area m^2  area_B=cabin_duct_area m^2
      settings: SourceProductBaseCode=SS  InternalSimscapePortConfiguration="{\"Bottom\":[],\"Left\":[{\"id\":\"A\",\"label\":\"A\",\"type\":\"foundation.moist_air.moist_air\"},{\"id\":\"V\",\"label\":\"V\",\"type\":\"input\"}],\"Right\":[{\"id\":\"B\",\"label\":\"B\",\"type\":\"foundation.moist_air.moist_air\"}],\"Top\":[]}"
  Fan Area [m^2] : Gain  Gain=fan_area
  Flow Resistance (2P) : fl_lib/Two-Phase Fluid/Elements/Flow Resistance (2P)  delta_p_nominal=1e-2 MPa  mdot_nominal=0.01 kg/s  v_nominal=0 m^3/kg  area=pi * refrigerant_pipe_D^2 / 4 m^2  laminar_fraction=1e-3
      settings: SourceProductBaseCode=SS  InternalSimscapePortConfiguration="{\"Bottom\":[],\"Left\":[{\"id\":\"A\",\"label\":\"A\",\"type\":\"foundation.two_phase_fluid.two_phase_fluid\"}],\"Right\":[{\"id\":\"B\",\"label\":\"B\",\"type\":\"foundation.two_phase_fluid.two_phase_fluid\"}],\"Top\":[]}"
  Max Fan : Gain  Gain=14.4
  Perfect Insulator : fl_lib/Thermal/Thermal Elements/Perfect Insulator  T_specify=off  T_priority=None  T=0 K  T_nominal_specify=off  T_nominal_unit=K  T_nominal_value=1
  Receiver : SimscapeFluids_lib/Two-Phase Fluid/Tanks & Accumulators/Receiver Accumulator (2P)  volume=2 l  area_AV=0.01 m^2  area_BV=0.01 m^2  area_AL=pi * refrigerant_pipe_D^2 / 4 m^2  area_BL=pi * refrigerant_pipe_D^2 / 4 m^2  V_frac_error=simscape.enum.assert.action.none  V_frac_min=0.05  V_frac_max=0.95  V_frac_smooth=0.05  p_crit_error=simscape.enum.assert.action.error  hc_vap=20 W/(m^2 * K)  hc_liq=100 W/(m^2 * K)  surface_area=0.06 m^2  receiver_accumulator_energy_spec=fluids.two_phase_fluid.enum.receiver_accumulator_energy_spec.volume_fraction  p_init=refrigerant_p_init MPa  T_init=293.15 K  M_frac_init=0.5  V_frac_init=1 - refrigerant_alpha_init  h_init=1500 kJ/kg  u_init=1500 kJ/kg  tau_vap_cond=1 s
      settings: SourceProductBaseCode=SH  InternalSimscapePortConfiguration="{\"Bottom\":[],\"Left\":[{\"id\":\"AV\",\"label\":\"AV\",\"type\":\"foundation.two_phase_fluid.two_phase_fluid\"},{\"id\":\"AL\",\"label\":\"AL\",\"type\":\"foundation.two_phase_fluid.two_phase_fluid\"},{\"id\":\"H\",\"label\":\"H\",\"type\":\"foundation.thermal.thermal\"}],\"Right\":[{\"id\":\"BV\",\"label\":\"BV\",\"type\":\"foundation.two_phase_fluid.two_phase_fluid\"},{\"id\":\"BL\",\"label\":\"BL\",\"type\":\"foundation.two_phase_fluid.two_phase_fluid\"},{\"id\":\"L\",\"label\":\"L\",\"type\":\"output\"}],\"Top\":[]}"
  Refrigerant Properties : SimscapeFluids_lib/Two-Phase Fluid/Utilities/Two-Phase Fluid Predefined Properties (2P)  fluid=fluids.two_phase_fluid.utilities.enum.Fluid.R134a  p_atm=0.101325 MPa  q_rev=0.01 Pa
      settings: SourceProductBaseCode=SH
  SR1 : Subsystem
      mask Display: disp(get_param(gcb, 'Name'))
  SR2 : Subsystem
      mask Display: disp(get_param(gcb, 'Name'))
  Simulink-PS Converter : nesl_utility/Simulink-PS Converter  PhysicalDomain=network_engine_domain  SubClassName=ps_input  LeftPortType=input  RightPortType=output  PseudoPeriodic=off  Frequencies=[]  NoiseDistribution=none  NoiseParameters=[]  Unit=m^3/s  AffineConversion=off  FilteringAndDerivatives=provide  SimscapeFilterOrder=1  InputFilterTimeConstant=0.001  UdotUserProvided=0
      settings: SourceProductBaseCode=PW,SS
  Simulink-PS Converter1 : nesl_utility/Simulink-PS Converter  PhysicalDomain=network_engine_domain  SubClassName=ps_input  LeftPortType=input  RightPortType=output  PseudoPeriodic=off  Frequencies=[]  NoiseDistribution=none  NoiseParameters=[]  Unit=degC  AffineConversion=on  FilteringAndDerivatives=provide  SimscapeFilterOrder=1  InputFilterTimeConstant=0.001  UdotUserProvided=0
      settings: SourceProductBaseCode=PW,SS
  Simulink-PS Converter5 : nesl_utility/Simulink-PS Converter  PhysicalDomain=network_engine_domain  SubClassName=ps_input  LeftPortType=input  RightPortType=output  PseudoPeriodic=off  Frequencies=[]  NoiseDistribution=none  NoiseParameters=[]  Unit=MPa  AffineConversion=off  FilteringAndDerivatives=provide  SimscapeFilterOrder=1  InputFilterTimeConstant=0.001  UdotUserProvided=0
      settings: SourceProductBaseCode=PW,SS
  Simulink-PS Converter6 : nesl_utility/Simulink-PS Converter  PhysicalDomain=network_engine_domain  SubClassName=ps_input  LeftPortType=input  RightPortType=output  PseudoPeriodic=off  Frequencies=[]  NoiseDistribution=none  NoiseParameters=[]  Unit=1  AffineConversion=off  FilteringAndDerivatives=provide  SimscapeFilterOrder=1  InputFilterTimeConstant=0.001  UdotUserProvided=0
      settings: SourceProductBaseCode=PW,SS
  Simulink-PS Converter7 : nesl_utility/Simulink-PS Converter  PhysicalDomain=network_engine_domain  SubClassName=ps_input  LeftPortType=input  RightPortType=output  PseudoPeriodic=off  Frequencies=[]  NoiseDistribution=none  NoiseParameters=[]  Unit=1  AffineConversion=off  FilteringAndDerivatives=provide  SimscapeFilterOrder=1  InputFilterTimeConstant=0.001  UdotUserProvided=0
      settings: SourceProductBaseCode=PW,SS
  Transfer Fcn : TransferFcn  Denominator=[5 1]
  A : PMIOPort  Side=Left
  T : PMIOPort  Port=2  Side=Left
  B : PMIOPort  Port=3  Side=Right
  wires:
  Max Fan/1 -> Air Speed Table [m/s]/2
  Air Speed Table [m/s]/1 -> Transfer Fcn/1
  [T_env] -> Simulink-PS Converter1/1
  [p_env] -> Simulink-PS Converter5/1
  [RH_env] -> Simulink-PS Converter6/1
  [CO2_env] -> Simulink-PS Converter7/1
  [cmd_fan] -> Max Fan/1
  [v_vehicle] -> Air Speed Table [m/s]/1
  Fan Area [m^2]/1 -> Simulink-PS Converter/1
  Transfer Fcn/1 -> Fan Area [m^2]/1
  connections:
  Condenser/LConn1 -- SR1/RConn1
  Condenser/LConn3 -- SR2/LConn1
  Receiver/LConn2 -- Flow Resistance (2P)/RConn1
  Cap (2P)/LConn1 -- Receiver/LConn1
  Cap (2P)1/LConn1 -- Receiver/RConn1
  Condenser/RConn1 -- T/RConn1
  Simulink-PS Converter5/RConn1 -- Environment Air/RConn2
  Simulink-PS Converter7/RConn1 -- Environment Air/RConn4
  Simulink-PS Converter6/RConn1 -- Environment Air/RConn3
  Simulink-PS Converter1/RConn1 -- Environment Air/RConn1
  Fan/RConn1 -- Environment Air/LConn1
  Fan/LConn1 -- Condenser/RConn3
  Fan/LConn2 -- Simulink-PS Converter/RConn1
  Perfect Insulator/LConn1 -- Receiver/LConn3
  SR1/LConn1 -- Refrigerant Properties/RConn1 -- A/RConn1
  SR2/RConn1 -- Flow Resistance (2P)/LConn1
  Receiver/RConn2 -- B/RConn1

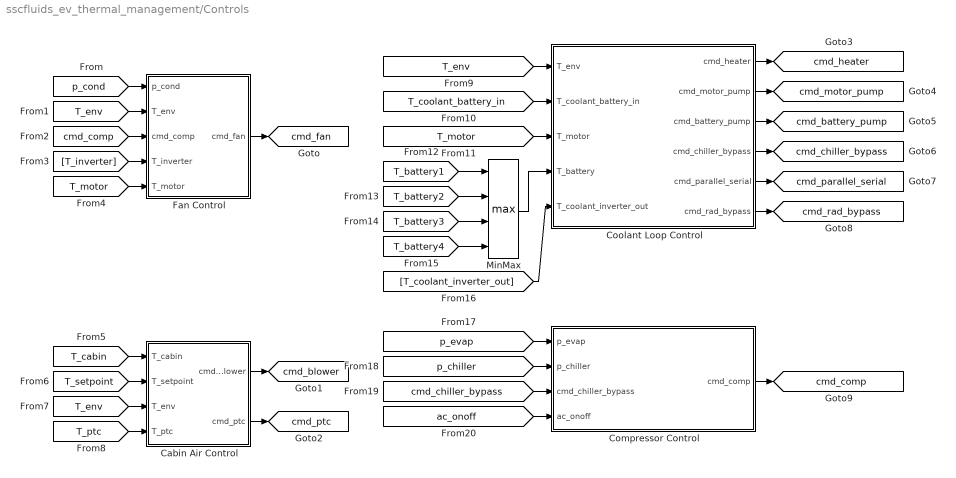
== system sscfluids_ev_thermal_management/Controls ==
  Cabin Air Control : Subsystem
  Compressor Control : Subsystem
  Coolant Loop Control : Subsystem
  Fan Control : Subsystem
  MinMax : MinMax  Function=max  Inputs=4
  tag scope: cmd_battery_pump=global, cmd_blower=global, cmd_chiller_bypass=global, cmd_comp=global, cmd_fan=global, cmd_heater=global, cmd_motor_pump=global, cmd_parallel_serial=global, cmd_ptc=global, cmd_rad_bypass=global
  wires:
  [p_cond] -> Fan Control/1(p_cond)
  [T_env] -> Fan Control/2(T_env)
  [T_inverter] -> Fan Control/4(T_inverter)
  [T_motor] -> Fan Control/5(T_motor)
  [T_env] -> Coolant Loop Control/1(T_env)
  [T_coolant_battery_in] -> Coolant Loop Control/2(T_coolant_battery_in)
  Fan Control/1(cmd_fan) -> [cmd_fan]
  Coolant Loop Control/1(cmd_heater) -> [cmd_heater]
  Coolant Loop Control/2(cmd_motor_pump) -> [cmd_motor_pump]
  Coolant Loop Control/3(cmd_battery_pump) -> [cmd_battery_pump]
  [p_evap] -> Compressor Control/1(p_evap)
  [p_chiller] -> Compressor Control/2(p_chiller)
  [cmd_chiller_bypass] -> Compressor Control/3(cmd_chiller_bypass)
  [ac_onoff] -> Compressor Control/4(ac_onoff)
  Compressor Control/1(cmd_comp) -> [cmd_comp]
  Cabin Air Control/1(cmd_blower) -> [cmd_blower]
  Cabin Air Control/2(cmd_ptc) -> [cmd_ptc]
  Coolant Loop Control/4(cmd_chiller_bypass) -> [cmd_chiller_bypass]
  Coolant Loop Control/5(cmd_parallel_serial) -> [cmd_parallel_serial]
  Coolant Loop Control/6(cmd_rad_bypass) -> [cmd_rad_bypass]
  [T_motor] -> Coolant Loop Control/3(T_motor)
  [T_battery3] -> MinMax/3
  [T_battery4] -> MinMax/4
  [T_battery2] -> MinMax/2
  [T_battery1] -> MinMax/1
  [T_coolant_inverter_out] -> Coolant Loop Control/5(T_coolant_inverter_out)
  MinMax/1 -> Coolant Loop Control/4(T_battery)
  [cmd_comp] -> Fan Control/3(cmd_comp)
  [T_cabin] -> Cabin Air Control/1(T_cabin)
  [T_setpoint] -> Cabin Air Control/2(T_setpoint)
  [T_env] -> Cabin Air Control/3(T_env)
  [T_ptc] -> Cabin Air Control/4(T_ptc)

== system sscfluids_ev_thermal_management/DCDC ==
  Controlled Heat Flow Rate Source : fl_lib/Thermal/Thermal Sources/Controlled Heat Flow Rate Source
  Coolant Jacket : SimscapeFluids_lib/Thermal Liquid/Pipes & Fittings/Pipe (TL)  dynamic_compressibility=1  inertia=0  num_segments=1  pipe_length=0.2 m  area=pi * coolant_channel_D^2 / 4 m^2  Dh=0.1128 m  wall_spec=1  Dh_rigid=coolant_channel_D m  wall_compliance=1.2e-6 m/MPa  wall_time_constant=0.01 s  elevation_spec=foundation.enum.constant_variable.constant  elevation_gain=0 m  g=9.81 m/s^2  pressure_loss_spec=1  length_add=0 m  roughness=1.5e-5 m  Re_friction_TLU=[ 400 1000 1.5e+3 3e+3 4e+3 6e+3 1e+4 2e+4 4e+4 6e+4 1e+5 1e+8 ]  friction_factor_TLU=[ 0.264 0.112 0.07099999999999999 0.0417 0.0387 0.0268 0.025 0.0232 0.0226 0.022 0.0214 0.0214 ]  shape_factor=64  Re_lam=100  Re_tur=500  mdot_nominal=[ 0.1 1 ] kg/s  p_diff_nominal=[ 0.001 0.01 ] MPa  mdot_threshold=1e-6 kg/s  heat_transfer_spec=4  mdot_nominal_heat=[ 0.1 1 ] kg/s  T_in_nominal=[ 293.15 293.15 ] K  T_out_nominal=[ 300 300 ] K  p_in_nominal_heat=[ 0.101325 0.101325 ] MPa  T_wall_nominal=[ 303.15 303.15 ] K  a_coeff=0.3  b_Re_power=0.8  c_Pr_power=0.33  Nu_lam=3.66  Re_Colburn_TLU=[ 100 150 1000 ]  Colburn_factor_TLU=[ 0.019 0.013 0.002 ]  Re_Nu_TLU=[ 100 150 1000 ]  Pr_Nu_TLU=[ 1 10 ]  Nu_TLU=[ 3.72 4.21; 3.75 4.44; 4.21 7.15 ]  T0_vec=coolant_T_init degC  p0_vec=coolant_p_init MPa  mdot0=0.1 kg/s
      settings: SourceProductBaseCode=SH
  DC-DC Converter : fl_lib/Thermal/Thermal Elements/Thermal Mass  mass=1 kg  sp_heat=447 J/kg/K  T_specify=on  T_priority=High  T=coolant_T_init degC  T_nominal_specify=off  T_nominal_unit=K  T_nominal_value=1  Q_specify=off  Q_priority=None  Q=0 W  Q_nominal_specify=off  Q_nominal_unit=W  Q_nominal_value=1
  Flow Resistance (TL) : fl_lib/Thermal Liquid/Elements/Flow Resistance (TL)  delta_p_nominal=2e-3 MPa  mdot_nominal=0.02 kg/s  area=pi * coolant_pipe_D^2 / 4 m^2  laminar_fraction=1e-3
      settings: SourceProductBaseCode=SS
  Flow Resistance (TL)1 : fl_lib/Thermal Liquid/Elements/Flow Resistance (TL)  delta_p_nominal=1e-5 MPa  mdot_nominal=0.02 kg/s  area=pi * coolant_pipe_D^2 / 4 m^2  laminar_fraction=1e-3
      settings: SourceProductBaseCode=SS
  PS-Simulink Converter : nesl_utility/PS-Simulink Converter  PhysicalDomain=network_engine_domain  SubClassName=ps_output  LeftPortType=input  RightPortType=output  PseudoPeriodic=off  Frequencies=[]  Unit=degC  AffineConversion=on
      settings: SourceProductBaseCode=PW,SS
  Simulink-PS Converter : nesl_utility/Simulink-PS Converter  PhysicalDomain=network_engine_domain  SubClassName=ps_input  LeftPortType=input  RightPortType=output  PseudoPeriodic=off  Frequencies=[]  NoiseDistribution=none  NoiseParameters=[]  Unit=W  AffineConversion=off  FilteringAndDerivatives=provide  SimscapeFilterOrder=1  InputFilterTimeConstant=0.001  UdotUserProvided=0
      settings: SourceProductBaseCode=PW,SS
  Temperature Sensor : fl_lib/Thermal/Thermal Sensors/Temperature Sensor
  Thermal Reference : fl_lib/Thermal/Thermal Elements/Thermal Reference
  Thermal Reference1 : fl_lib/Thermal/Thermal Elements/Thermal Reference
  B : PMIOPort  Side=Left
  A : PMIOPort  Port=2  Side=Right
  tag scope: T_dcdc=global
  wires:
  [Q_dcdc] -> Simulink-PS Converter/1
  PS-Simulink Converter/1 -> [T_dcdc]
  connections:
  Controlled Heat Flow Rate Source/LConn1 -- DC-DC Converter/LConn1 -- Coolant Jacket/LConn2 -- Temperature Sensor/LConn1
  Simulink-PS Converter/RConn1 -- Controlled Heat Flow Rate Source/RConn1
  Controlled Heat Flow Rate Source/RConn2 -- Thermal Reference/LConn1
  Thermal Reference1/LConn1 -- Temperature Sensor/RConn1
  Temperature Sensor/RConn2 -- PS-Simulink Converter/LConn1
  Coolant Jacket/LConn1 -- Flow Resistance (TL)/RConn1
  Coolant Jacket/RConn1 -- Flow Resistance (TL)1/LConn1
  Flow Resistance (TL)/LConn1 -- A/RConn1
  Flow Resistance (TL)1/RConn1 -- B/RConn1
